simulink model "lr_8_slx"  (R2018a)
settings: Solver=FixedStepAuto  StartTime=0.0  StopTime=0.1  FixedStep=0.1/10240  RelTol=1e-3
libraries: dsparch4 x3
settings Model: Creator=Asus  LastModifiedBy=Asus

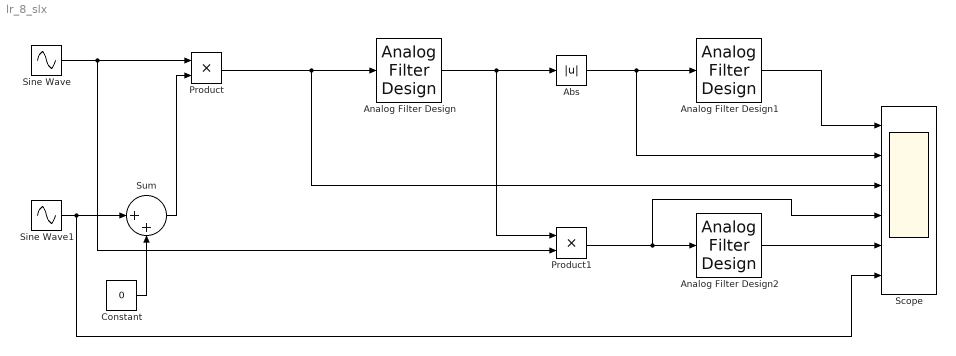
== system lr_8_slx ==
  Abs : Abs
  Analog Filter Design : dsparch4/Analog Filter Design  method=Butterworth  filttype=Bandpass  N=8  Wlo=600*2*pi  Whi=1400*2*pi  Rp=2  Rs=40
  Analog Filter Design1 : dsparch4/Analog Filter Design  method=Butterworth  filttype=Lowpass  N=8  Wlo=800*2*pi  Whi=80  Rp=2  Rs=40
  Analog Filter Design2 : dsparch4/Analog Filter Design  method=Butterworth  filttype=Lowpass  N=8  Wlo=100*2*pi  Whi=80  Rp=2  Rs=40
  Constant : Constant  Value=0
  Product : Product
  Product1 : Product
  Scope : Scope  NumInputPorts=6
  Sine Wave : Sin  Frequency=1000*2*pi  SampleTime=0
  Sine Wave1 : Sin  Frequency=100*2*pi  SampleTime=0
  Sum : Sum  Inputs=|++
  wires:
  Sine Wave/1 -> Product1/2, Product/1
  Constant/1 -> Sum/2
  Sine Wave1/1 -> Scope/6, Sum/1
  Sum/1 -> Product/2
  Product/1 -> Scope/3, Analog Filter Design/1
  Analog Filter Design/1 -> Product1/1, Abs/1
  Abs/1 -> Scope/2, Analog Filter Design1/1
  Analog Filter Design1/1 -> Scope/1
  Analog Filter Design2/1 -> Scope/5
  Product1/1 -> Scope/4, Analog Filter Design2/1
